simulink model "modello_adattativo"  (R2024a)
settings: Solver=VariableStepAuto  StartTime=0.0  StopTime=70  RelTol=1e-3
model workspace (MAT data in the model file):
  q0 = [0.785398163397; 0.523598775598; 0.628318530718; 0.5]
values from neighbouring files (symbols this model uses):
  Kd = diag([108 68 58 200])    [TRAIETTORIA.m]    (also in traiettoriafperfettadefinitiva1.m)
  Kp = diag([13 13 11 1000])    [TRAIETTORIA.m]    (also in traiettoriafperfettadefinitiva1.m)
  PI0 = [ml1; Il1; Im1; Fm1; ml2; Il2; Im2; Fm2; ml3; Im3; Fm3;ml4; Il4; Im4; Fm4]    [traiettoriafperfettadefinitiva1.m]
undefined symbols (not defined in the file or in its folder): DiscIntNeverNeededParam
settings Model: Creator=ThinkPad  LastModifiedBy=UTENTE
settings ModelReferenceCC: EnableRefExpFcnMdlSchedulingChecks=on
settings RTWCC: GPUComputeCapability=3.5

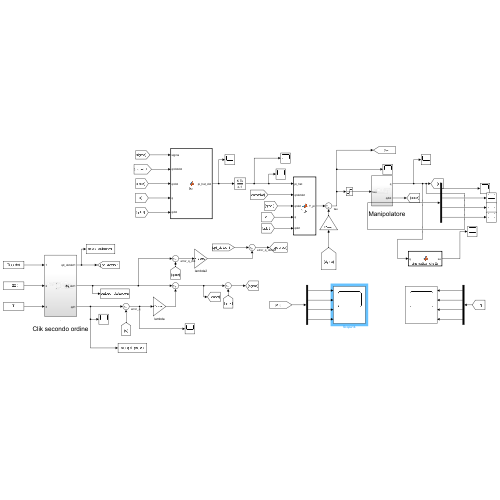
[thumbnail: Simulink's stored preview of the top-level diagram]
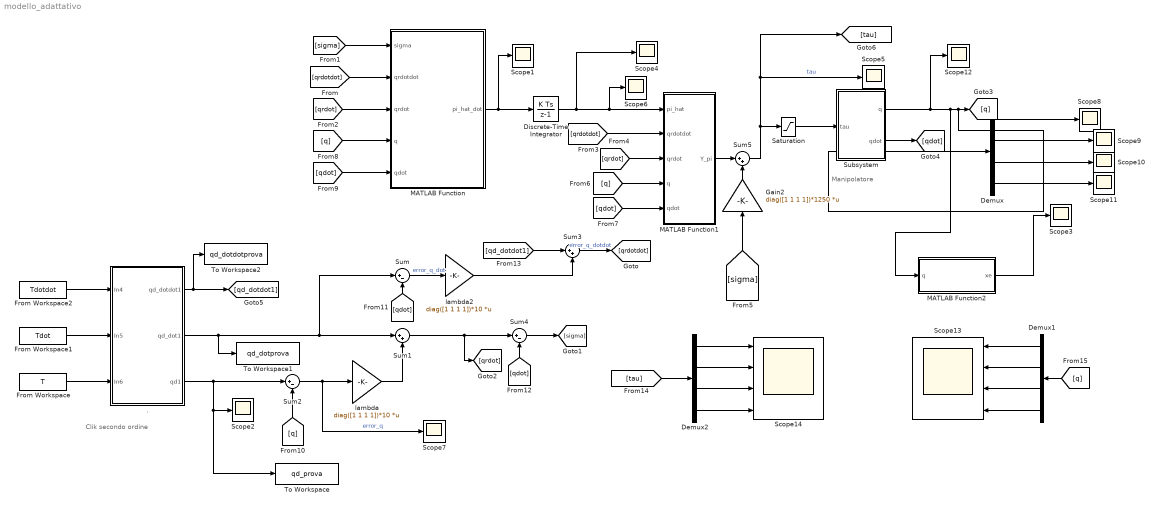
== system modello_adattativo ==
  note: Clik secondo ordine
  note: Manipolatore
  . : Subsystem
  Demux : Demux
  Demux1 : Demux
  Demux2 : Demux
  Discrete-Time Integrator : DiscreteIntegrator  InitialCondition=PI0  SampleTime=0.001  ICPrevOutput=DiscIntNeverNeededParam  ICPrevScaledInput=DiscIntNeverNeededParam
  From Workspace : FromWorkspace  VariableName=T  SampleTime=0.001
  From Workspace1 : FromWorkspace  VariableName=Tdot  SampleTime=0.001
  From Workspace2 : FromWorkspace  VariableName=Tdotdot  SampleTime=0.001
  Gain2 : Gain  Gain=diag([1 1 1 1])*1250  Multiplication=Matrix(K*u) (u vector)
  MATLAB Function : MATLAB Function  TreatAsAtomicUnit=on
  MATLAB Function1 : MATLAB Function  TreatAsAtomicUnit=on
  MATLAB Function2 : MATLAB Function  TreatAsAtomicUnit=on
  Saturation : Saturate  UpperLimit=1000  LowerLimit=-1000
  Scope{1..12} (12 alike) : Scope
  Scope13 : Scope  NumInputPorts=4
  Scope14 : Scope  NumInputPorts=4
  Subsystem : Subsystem
  Sum : Sum  Inputs=|+-
  Sum1 : Sum  Inputs=|++
  Sum2 : Sum  Inputs=|+-
  Sum3 : Sum  Inputs=|++
  Sum4 : Sum  Inputs=|+-
  Sum5 : Sum  Inputs=|++
  To Workspace : ToWorkspace  VariableName=qd_prova  SampleTime=0.001
  To Workspace1 : ToWorkspace  VariableName=qd_dotprova  SampleTime=0.001
  To Workspace2 : ToWorkspace  VariableName=qd_dotdotprova  SampleTime=0.001
  lambda : Gain  Gain=diag([1 1 1 1])*10  Multiplication=Matrix(K*u) (u vector)
  lambda2 : Gain  Gain=diag([1 1 1 1])*10  Multiplication=Matrix(K*u) (u vector)
  wires:
  From Workspace/1 -> ./3(In6)
  Subsystem/1(q) -> Scope12/1, MATLAB Function2/1(q), Demux/1, [q]
  [sigma] -> Gain2/1
  Demux2/3 -> Scope14/3
  Demux2/4 -> Scope14/4
  MATLAB Function1/1(Y_pi) -> Sum5/1
  Demux1/3 -> Scope13/3
  [q] -> MATLAB Function/4(q)
  Demux2/2 -> Scope14/2
  [qdot] -> Sum/2
  Demux1/2 -> Scope13/2
  Demux1/4 -> Scope13/4
  [qdot] -> MATLAB Function/5(qdot)
  Demux1/1 -> Scope13/1
  [sigma] -> MATLAB Function/1(sigma)
  [qdot] -> Sum4/2
  ./3(qd1) -> To Workspace/1, Scope2/1, Sum2/1
  Demux/3 -> Scope10/1
  Sum1/1 -> Sum4/1, [qrdot]
  [qrdotdot] -> MATLAB Function1/2(qrdotdot)
  [qrdotdot] -> MATLAB Function/2(qrdotdot)
  Demux2/1 -> Scope14/1
  Demux/2 -> Scope9/1
  Sum3/1 -> [qrdotdot]  "error_q_dotdot"
  Discrete-Time Integrator/1 -> Scope4/1, Scope6/1, MATLAB Function1/1(pi_hat)
  From Workspace2/1 -> ./1(In4)
  MATLAB Function2/1(xe) -> Scope3/1
  [q] -> Sum2/2
  [qdot] -> MATLAB Function1/5(qdot)
  From Workspace1/1 -> ./2(In5)
  Sum2/1 -> lambda/1, Scope7/1  "error_q"
  lambda2/1 -> Sum3/2
  Gain2/1 -> Sum5/2
  Sum5/1 -> Saturation/1, [tau], Scope5/1  "tau"
  MATLAB Function/1(pi_hat_dot) -> Discrete-Time Integrator/1, Scope1/1
  [qrdot] -> MATLAB Function/3(qrdot)
  Sum4/1 -> [sigma]
  ./1(qd_dotdot1) -> To Workspace2/1, [qd_dotdot1]
  Demux/4 -> Scope11/1
  Subsystem/2(qdot) -> [qdot]
  Sum/1 -> lambda2/1  "error_q_dot"
  [q] -> MATLAB Function1/4(q)
  lambda/1 -> Sum1/2
  ./2(qd_dot1) -> To Workspace1/1, Sum/1, Sum1/1
  Demux/1 -> Scope8/1
  [qrdot] -> MATLAB Function1/3(qrdot)
  [qd_dotdot1] -> Sum3/1
  [tau] -> Demux2/1
  [q] -> Demux1/1
  Saturation/1 -> Subsystem/1(tau)

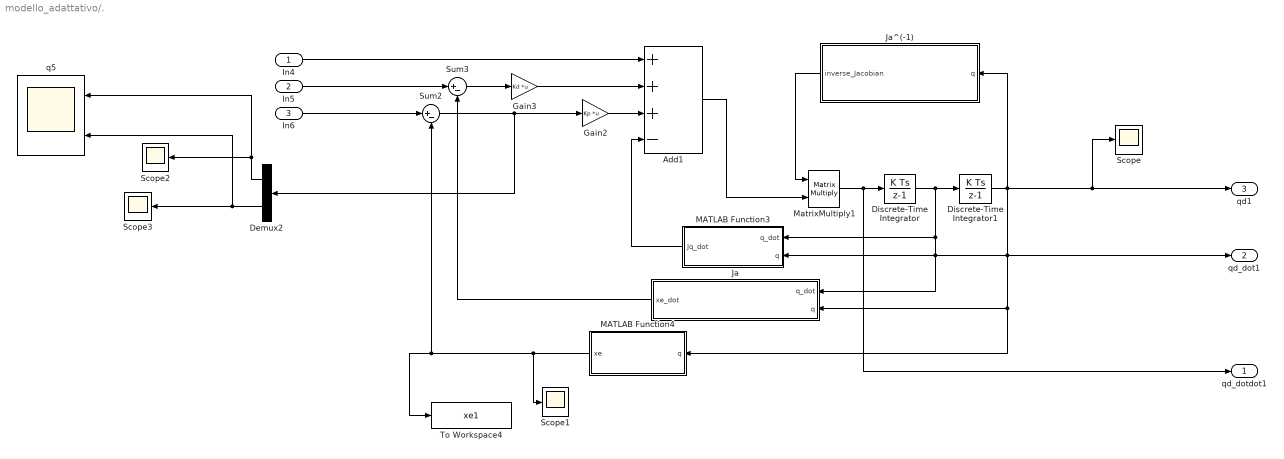
== system modello_adattativo/. ==
  In4 : Inport
  In5 : Inport  Port=2
  In6 : Inport  Port=3
  Add1 : Sum  Inputs=+++-
  Demux2 : Demux  Outputs=[3 1]
  Discrete-Time Integrator : DiscreteIntegrator  InitialCondition=[0 0 0 0]'  SampleTime=0.001  ICPrevOutput=DiscIntNeverNeededParam  ICPrevScaledInput=DiscIntNeverNeededParam
  Discrete-Time Integrator1 : DiscreteIntegrator  InitialCondition=q0  SampleTime=0.001  ICPrevOutput=DiscIntNeverNeededParam  ICPrevScaledInput=DiscIntNeverNeededParam
  Gain2 : Gain  Gain=Kp  Multiplication=Matrix(K*u)
  Gain3 : Gain  Gain=Kd  Multiplication=Matrix(K*u)
  Ja : MATLAB Function  TreatAsAtomicUnit=on
  Ja^(-1) : MATLAB Function  TreatAsAtomicUnit=on
  MATLAB Function3 : MATLAB Function  TreatAsAtomicUnit=on
  MATLAB Function4 : MATLAB Function  TreatAsAtomicUnit=on
  MatrixMultiply1 : Product  Multiplication=Matrix(*)
  Scope{,1..3} (4 alike) : Scope
  Sum2 : Sum  Inputs=|+-
  Sum3 : Sum  Inputs=|+-
  To Workspace4 : ToWorkspace  VariableName=xe1  SampleTime=0.001
  q5 : Scope  NumInputPorts=2
  qd_dotdot1 : Outport
  qd_dot1 : Outport  Port=2
  qd1 : Outport  Port=3
  wires:
  Discrete-Time Integrator1/1 -> Scope/1, qd1/1, Ja/2(q), MATLAB Function4/1(q), MATLAB Function3/2(q), Ja^(-1)/1(q)
  MatrixMultiply1/1 -> qd_dotdot1/1, Discrete-Time Integrator/1
  Sum3/1 -> Gain3/1
  MATLAB Function3/1(Jq_dot) -> Add1/4
  Ja/1(xe_dot) -> Sum3/2
  Ja^(-1)/1(inverse_Jacobian) -> MatrixMultiply1/1
  Add1/1 -> MatrixMultiply1/2
  MATLAB Function4/1(xe) -> Scope1/1, To Workspace4/1, Sum2/2
  Discrete-Time Integrator/1 -> Ja/1(q_dot), qd_dot1/1, MATLAB Function3/1(q_dot), Discrete-Time Integrator1/1
  Gain3/1 -> Add1/2
  In4/1 -> Add1/1
  In6/1 -> Sum2/1
  In5/1 -> Sum3/1
  Gain2/1 -> Add1/3
  Demux2/2 -> q5/2, Scope3/1
  Sum2/1 -> Demux2/1, Gain2/1
  Demux2/1 -> q5/1, Scope2/1

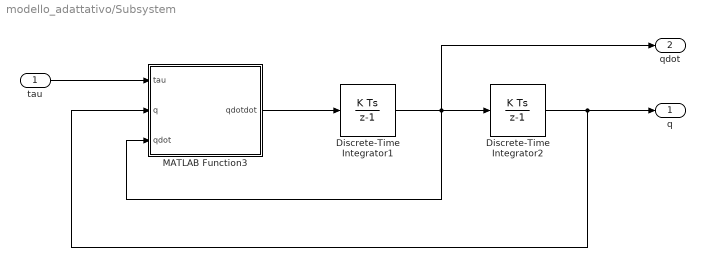
== system modello_adattativo/Subsystem ==
  tau : Inport
  Discrete-Time Integrator1 : DiscreteIntegrator  InitialCondition=[0 0 0 0]'  SampleTime=0.001  ICPrevOutput=DiscIntNeverNeededParam  ICPrevScaledInput=DiscIntNeverNeededParam
  Discrete-Time Integrator2 : DiscreteIntegrator  InitialCondition=[pi/4,pi/6,pi/5,0.5]'  SampleTime=0.001  ICPrevOutput=DiscIntNeverNeededParam  ICPrevScaledInput=DiscIntNeverNeededParam
  MATLAB Function3 : MATLAB Function  TreatAsAtomicUnit=on
  q : Outport
  qdot : Outport  Port=2
  wires:
  Discrete-Time Integrator2/1 -> q/1, MATLAB Function3/2(q)
  Discrete-Time Integrator1/1 -> qdot/1, Discrete-Time Integrator2/1, MATLAB Function3/3(qdot)
  tau/1 -> MATLAB Function3/1(tau)
  MATLAB Function3/1(qdotdot) -> Discrete-Time Integrator1/1

== matlab function modello_adattativo/Subsystem/MATLAB Function3 ==
  data: tau input; q input; qdot input; qdotdot output
function qdotdot = fcn(tau, q, qdot)
    d0=1; %m
    a1=0.5; %m
    a2=0.5; %m
    
    l1=0.25; %m
    l2=0.25; %m
    ml1=20; %kg
    ml2=20; %kg
    ml3=10; %kg
    ml4=0; %kg
    Il1=4; %kg�m2
    Il2=4; %kg�m2
    Il3=0;
    Il4=1; %kg�m2
    Kr1=1;
    Kr2=1;
    Kr3=50; %rad/m
    Kr4 =20;
    Im1=0.01; %kg�m2
    Im2=0.01; %kg�m2
    Im3=0.005; %kg�m2
    Im4=0.001;%kg
    Fm1=0.00005; %N�m�s/rad
    Fm2=0.00005; %N�m�s/rad
    Fm3=0.01; %N�m�s/rad
    Fm4 =0.005; %N�m�s/rad
    mm1=0;
    mm2=0;
    mm3=0;
    mm4=0;
    ml=3;
    
    Jp_l1=[-l1*sin(q(1)) 0 0 0; 
            l1*cos(q(1)) 0 0 0; 
            0 0 0 0];
    Jo_l1=[zeros(2,4)
           1 0 0 0];
    
    Jp_l2=[-a1*sin(q(1))-l2*sin(q(1)+q(2)) -l2*sin(q(1)+q(2)) 0 0; 
            a1*cos(q(1))+l2*cos(q(1)+q(2)) l2*cos(q(1)+q(2)) 0 0;
            0 0 0 0];
    Jo_l2=[zeros(2,4)
           1 1 0 0];
    
    Jp_l3=[-a1*sin(q(1))-a2*sin(q(1)+q(2)) -a2*sin(q(1)+q(2)) 0 0; 
            a1*cos(q(1))+a2*cos(q(1)+q(2)) a2*cos(q(1)+q(2)) 0 0;
            0 0 -1 0];
    Jo_l3 = [zeros(2,4)
             1 1 0 0];
    
    Jp_l4=Jp_l3;
    Jo_l4 = [zeros(2,4)
             1 1 0 -1];
    
    Jp_m1 = [0 0 0 0;
             0 0 0 0;
             0 0 0 0];
    Jo_m1 = [zeros(2,4)
             Kr1 0 0 0];
    
    Jp_m2 = [-a1*sin(q(1)) 0 0 0; 
            a1*cos(q(1)) 0 0 0; 
            0 0 0 0];
    Jo_m2 = [zeros(2,4)
             1 Kr2 0 0];
    
    Jp_m3 = [-a1*sin(q(1))-a2*sin(q(1)+q(2)) -a2*sin(q(1)+q(2)) 0 0; 
              a1*cos(q(1))+a2*cos(q(1)+q(2)) a2*cos(q(1)+q(2)) 0 0;
              0 0 0 0];
    Jo_m3 = [zeros(2,4)
             1 1 -Kr3 0];
    
    Jp_m4 = [-a1*sin(q(1))-a2*sin(q(1)+q(2)) -a2*sin(q(1)+q(2)) 0 0; 
              a1*cos(q(1))+a2*cos(q(1)+q(2)) a2*cos(q(1)+q(2)) 0 0;
              0 0 -1 0];
    Jo_m4 = [zeros(2,4)
             1 1 0 -Kr4];
    B1 = ml1*Jp_l1'*Jp_l1+Jo_l1'*Il1*Jo_l1+mm1*Jp_m1'*Jp_m1+Jo_m1'*Im1*Jo_m1;
    B2 = ml2*Jp_l2'*Jp_l2+Jo_l2'*Il2*Jo_l2+mm2*Jp_m2'*Jp_m2+Jo_m2'*Im2*Jo_m2;
    B3 = ml3*Jp_l3'*Jp_l3+Jo_l3'*Il3*Jo_l3+mm3*Jp_m3'*Jp_m3+Jo_m3'*Im3*Jo_m3;
    B4 = (ml4+ml)*Jp_l4'*Jp_l4+Jo_l4'*Il4*Jo_l4+mm4*Jp_m4'*Jp_m4+Jo_m4'*Im4*Jo_m4;
    B = B1+B2+B3+B4;
    
    Fv = diag([Kr1^2*Fm1 Kr2^2*Fm2 Kr3^2*Fm3 Kr4^2*Fm4]);
    g=[0 0 -9.81*(ml+ml3) 0]';
    
Jpl1_dq1=[-l1*cos(q(1)) 0 0 0;
    -l1*sin(q(1)) 0 0 0;
    0 0 0 0];

Jpl2_dq1=[-a1*cos(q(1))-l2*cos(q(1)+q(2)) -l2*cos(q(1)+q(2)) 0 0;
    -a1*sin(q(1))-l2*sin(q(1)+q(2)) -l2*sin(q(1)+q(2)) 0 0;
    0 0 0 0];

Jpl2_dq2=[-a2*cos(q(1)+q(2)) -a2*cos(q(1)+q(2)) 0 0;
    -a2*sin(q(1)+q(2)) -a2*sin(q(1)+q(2)) 0 0;
    0 0 0 0];

Jpl4_dq1=[-a1*cos(q(1))-a2*cos(q(1)+q(2)) -a2*cos(q(1)+q(2)) 0 0;
    -a1*sin(q(1))-a2*sin(q(1)+q(2)) -a2*sin(q(1)+q(2)) 0 0;
    0 0 0 0];

Jpl4_dq2=[-a2*sin(q(1)+q(2)) -a2*sin(q(1)+q(2)) 0 0;
    -a2*cos(q(1)+q(2)) -a2*cos(q(1)+q(2)) 0 0;
    0 0 0 0];

% Calcolo matrice differenziate rispetto a dq1 dq2
dBdq1=ml1*(Jpl1_dq1'*Jp_l1+Jp_l1'*Jpl1_dq1)+ml2*(Jpl2_dq1'*Jp_l2+Jp_l2'*Jpl2_dq1)...
    +ml3*(Jpl4_dq1'*Jp_l4+Jp_l4'*Jpl4_dq1);

dBdq2=ml2*(Jpl2_dq2'*Jp_l2+Jp_l2'*Jpl2_dq2)+ml3*(Jpl4_dq2'*Jp_l4+Jp_l4'*Jpl4_dq2);

H=zeros(4,4,4);

% Inizializzazione simboli cristoffel del primo tipo
for i=1:4
    for j=1:4
        for k=1:4
            H(i,j,k)=0;
        end
    end
end

H(1,1,2)=1/2*(dBdq2(1,1)+dBdq1(1,2)-dBdq1(1,2));
H(1,2,1)=H(1,1,2); 
H(1,2,2)=1/2*(dBdq2(1,2)+dBdq2(1,2)-dBdq1(2,2));
H(2,1,1)=1/2*(dBdq1(2,1)+dBdq1(2,1)-dBdq2(1,1));
H(2,1,2)=1/2*(dBdq2(2,1)+dBdq1(2,2)-dBdq2(1,2));
H(2,2,1)=H(2,1,2);
H(2,2,2)=1/2*(dBdq2(2,2)+dBdq2(2,2)-dBdq2(2,2));


% C=sym('C',[4,4]);
C=zeros(4,4);
for i=1:4
    for j=1:4
        C(i,j)=0;
    end
end

% qdot=sym('qdot',[4,1]);

for i=1:4
    for j=1:4
        for k=1:4
            r=H(i,j,k)*qdot(k);
            C(i,j)=C(i,j)+r;
        end
    end
end

    
qdotdot = inv(B)*(tau-C*qdot-Fv*qdot-g);
end

== matlab function modello_adattativo/MATLAB Function ==
  data: sigma input; qrdotdot input; qrdot input; pi_hat_dot output; q input; qdot input
function pi_hat_dot = fcn(sigma, qrdotdot,qrdot,q,qdot)

d0=1; 
a1=0.5; 
a2=0.5;    
l1=0.25;
l2=0.25;
ml1=20; 
ml2=20; 
ml3=10; 
ml4=0; 
Il1=4; 
Il2=4; 
Il3=0;
Il4=1; 
kr1=1;
kr2=1;
kr3=50;
kr4 =20;
Im1=0.01;
Im2=0.01;
Im3=0.005;
Im4=0.001;
Fm1=0.00005;
Fm2=0.00005;
Fm3=0.01;
Fm4 =0.005;
mm1=0;
mm2=0;
mm3=0;
mm4=0;
ml=3;
    
pi = [ml1; Il1; Im1; Fm1; ml2; Il2; Im2; Fm2; ml3; Im3; Fm3;ml4; Il4; Im4; Fm4];
%Kpi=diag([650 500 500 500 650 500 150 500 200 850 200 0.1 650 1500 650]);

%Kpi=diag([3000 3000 3000 3000 3000 3000 3000 300 100 100 100 0.01 300 300 300]);
%Kpi=diag([1 1 1 1 1 1 1 1 1 1 1 0.01 1 1 1]*50);
Kpi=diag([500 500 500 500 500 500 500 500 500 50 500 0.01 500 500 500]);

qr1_dd = qrdotdot(1);
qr2_dd = qrdotdot(2);
qr3_dd = qrdotdot(3);
qr4_dd = qrdotdot(4);
qr1_d = qrdot(1);
qr2_d = qrdot(2);
qr3_d = qrdot(3);
qr4_d = qrdot(4);
q1 = q(1);
q2 = q(2);
q1_d = qdot(1);
q2_d = qdot(2);

% Y =[qrdotdot(1)*((cos(conj(q(1)))*cos(q(1)))/16 + (sin(conj(q(1)))*sin(q(1)))/16), qrdotdot(1), qrdotdot(1), qrdot(1), qrdotdot(2)*(cos(q(1) + q(2) - conj(q(1)) - conj(q(2)))/16 + cos(q(1) + q(2) - conj(q(1)))/8) + qrdotdot(1)*((cos(q(1) + q(2))/4 + cos(q(1))/2)*(cos(conj(q(1)))/2 + cos(conj(q(1)) + conj(q(2)))/4) + (sin(q(1) + q(2))/4 + sin(q(1))/2)*(sin(conj(q(1)))/2 + sin(conj(q(1)) + conj(q(2)))/4)), qrdotdot(1) + qrdotdot(2), qrdotdot(1) + qrdotdot(2), 0, qrdotdot(2)*(cos(q(1) + q(2) - conj(q(1)) - conj(q(2)))/4 + cos(q(1) + q(2) - conj(q(1)))/4) + qrdotdot(1)*((cos(q(1) + q(2))/2 + cos(q(1))/2)*(cos(conj(q(1)))/2 + cos(conj(q(1)) + conj(q(2)))/2) + (sin(q(1) + q(2))/2 + sin(q(1))/2)*(sin(conj(q(1)))/2 + sin(conj(q(1)) + conj(q(2)))/2)), qrdotdot(1) + qrdotdot(2) - 50*qrdotdot(3), 0, qrdotdot(1) + qrdotdot(2) - qrdotdot(4), qrdotdot(1) + qrdotdot(2) - 20*qrdotdot(4), 0;
% 0, 0, 0, 0, qrdotdot(1)*((cos(conj(q(1)) + conj(q(2)))*(cos(q(1) + q(2))/4 + cos(q(1))/2))/4 + (sin(conj(q(1)) + conj(q(2)))*(sin(q(1) + q(2))/4 + sin(q(1))/2))/4) + (qrdotdot(2)*cos(q(1) + q(2) - conj(q(1)) - conj(q(2))))/16, qrdotdot(1) + qrdotdot(2), qrdotdot(1) + qrdotdot(2), qrdot(2), qrdotdot(1)*((cos(conj(q(1)) + conj(q(2)))*(cos(q(1) + q(2))/2 + cos(q(1))/2))/2 + (sin(conj(q(1)) + conj(q(2)))*(sin(q(1) + q(2))/2 + sin(q(1))/2))/2) + (qrdotdot(2)*cos(q(1) + q(2) - conj(q(1)) - conj(q(2))))/4, qrdotdot(1) + qrdotdot(2) - 50*qrdotdot(3), 0, qrdotdot(1) + qrdotdot(2) - qrdotdot(4), qrdotdot(1) + qrdotdot(2) - 20*qrdotdot(4), 0;
% 0, 0, 0, 0, 0, 0, 0, 0, qrdotdot(3) - 981/100, 2500*qrdotdot(3) - 50*qrdotdot(2) - 50*qrdotdot(1), 2500*qrdot(3), 0, 0, 0;
% 0, 0, 0, 0, 0, 0, 0, 0, 0, 0, 0, qrdotdot(4) - qrdotdot(2) - qrdotdot(1), 400*qrdotdot(4) - 20*qrdotdot(2) - 20*qrdotdot(1), 400*qrdot(4)];
 

% Y =[l1^2*qrdotdot(1)*cos(q(1) - conj(q(1))), qrdotdot(1), kr1^2*qrdotdot(1), kr1^2*qrdot(1), l2^2*qrdotdot(1)*cos(q(1) + q(2) - conj(q(1)) - conj(q(2))) + l2^2*qrdotdot(2)*cos(q(1) + q(2) - conj(q(1)) - conj(q(2))) + a1^2*qrdotdot(1)*cos(q(1) - conj(q(1))) + a1*l2*qrdotdot(1)*cos(q(1) + q(2) - conj(q(1))) + a1*l2*qrdotdot(2)*cos(q(1) + q(2) - conj(q(1))) - (a1*a2*qrdot(2)*sin(q(1) + q(2) - conj(q(1))))/2 + a1*l2*qrdotdot(1)*cos(conj(q(1)) - q(1) + conj(q(2))) - (a1*a2*qrdot(2)*sin(conj(q(1)) - q(1) + conj(q(2))))/2, qrdotdot(1) + qrdotdot(2),       qrdotdot(1) + kr2*qrdotdot(2),            0, a2^2*qrdotdot(1)*cos(q(1) + q(2) - conj(q(1)) - conj(q(2))) - a2^2*qrdot(2)*cos(2*real(q(1)) + 2*real(q(2))) + a2^2*qrdotdot(2)*cos(q(1) + q(2) - conj(q(1)) - conj(q(2))) + a1^2*qrdotdot(1)*cos(q(1) - conj(q(1))) - (a1*a2*qrdot(2)*cos(2*real(q(1)) + conj(q(2))))/2 + a1*a2*qrdotdot(1)*cos(q(1) + q(2) - conj(q(1))) + a1*a2*qrdotdot(2)*cos(q(1) + q(2) - conj(q(1))) + a1*a2*qrdotdot(1)*cos(conj(q(1)) - q(1) + conj(q(2))) - (a1*a2*qrdot(2)*cos(q(2) + 2*real(q(1))))/2,           qrdotdot(1) + qrdotdot(2) - kr3*qrdotdot(3),            0, qrdotdot(1) + qrdotdot(2) - qrdotdot(4),           qrdotdot(1) + qrdotdot(2) - kr4*qrdotdot(4),            0;
%                                 0,         0,               0,            0,                                                                                                                                                                                                                     l2^2*qrdotdot(1)*cos(q(1) + q(2) - conj(q(1)) - conj(q(2))) + l2^2*qrdotdot(2)*cos(q(1) + q(2) - conj(q(1)) - conj(q(2))) + a1*l2*qrdotdot(1)*cos(conj(q(1)) - q(1) + conj(q(2))), qrdotdot(1) + qrdotdot(2), qrdotdot(2)*kr2^2 + qrdotdot(1)*kr2, kr2^2*qrdot(2),                                                                                                                                                                                                                                                          a2^2*qrdotdot(1)*cos(q(1) + q(2) - conj(q(1)) - conj(q(2))) + a2^2*qrdotdot(2)*cos(q(1) + q(2) - conj(q(1)) - conj(q(2))) + a1*a2*qrdotdot(1)*cos(conj(q(1)) - q(1) + conj(q(2))),           qrdotdot(1) + qrdotdot(2) - kr3*qrdotdot(3),            0, qrdotdot(1) + qrdotdot(2) - qrdotdot(4),           qrdotdot(1) + qrdotdot(2) - kr4*qrdotdot(4),            0;
%                                 0,         0,               0,            0,                                                                                                                                                                                                                                                                                                                                                                         0,                     0,                               0,            0,                                                                                                                                                                                                                                                                                                                                                                                            qrdotdot(3) - 981/100, kr3^2*qrdotdot(3) - kr3*qrdotdot(2) - kr3*qrdotdot(1), kr3^2*qrdot(3),                                 0,                                               0,            0;
%                                0,         0,               0,            0,                                                                                                                                                                                                                                                                                                                                                                         0,                     0,                               0,            0,                                                                                                                                                                                                                                                                                                                                                                                                              0,                                               0,            0, qrdotdot(4) - qrdotdot(2) - qrdotdot(1), kr4^2*qrdotdot(4) - kr4*qrdotdot(2) - kr4*qrdotdot(1), kr4^2*qrdot(4)];
%  
Y= [qr1_dd*(cos(q1)^2/16 + sin(q1)^2/16), qr1_dd, qr1_dd, qr1_d, qr1_dd*((sin(q1 + q2)/4 + sin(q1)/2)^2 + (cos(q1 + q2)/4 + cos(q1)/2)^2) - qr2_d*(q1_d*((sin(q1 + q2)*(cos(q1 + q2)/4 + cos(q1)/2))/2 - (cos(q1 + q2)*(sin(q1 + q2)/4 + sin(q1)/2))/2) + q2_d*((sin(q1 + q2)*(cos(q1 + q2)/4 + cos(q1)/2))/2 - (cos(q1 + q2)*(sin(q1 + q2)/4 + sin(q1)/2))/2)) + qr2_dd*((cos(q1 + q2)*(cos(q1 + q2)/4 + cos(q1)/2))/4 + (sin(q1 + q2)*(sin(q1 + q2)/4 + sin(q1)/2))/4) - q1_d*qr1_d*((sin(q1 + q2)*(cos(q1 + q2)/4 + cos(q1)/2))/2 - (cos(q1 + q2)*(sin(q1 + q2)/4 + sin(q1)/2))/2), qr1_dd + qr2_dd, qr1_dd + qr2_dd,     0, qr1_dd*((sin(q1 + q2)/2 + sin(q1)/2)^2 + (cos(q1 + q2)/2 + cos(q1)/2)^2) - qr2_d*(q2_d*(cos(q1 + q2)^2/4 - sin(q1 + q2)^2/4 + (cos(q1 + q2)*(cos(q1 + q2)/2 + cos(q1)/2))/2 - (sin(q1 + q2)*(sin(q1 + q2)/2 + sin(q1)/2))/2) + q1_d*((cos(q1 + q2)*(cos(q1 + q2)/2 + cos(q1)/2))/2 - (sin(q1 + q2)*(sin(q1 + q2)/2 + sin(q1)/2))/2)) + qr2_dd*((cos(q1 + q2)*(cos(q1 + q2)/2 + cos(q1)/2))/2 + (sin(q1 + q2)*(sin(q1 + q2)/2 + sin(q1)/2))/2) - q1_d*qr1_d*((cos(q1 + q2)*(cos(q1 + q2)/2 + cos(q1)/2))/2 - (sin(q1 + q2)*(sin(q1 + q2)/2 + sin(q1)/2))/2),         qr1_dd + qr2_dd - 50*qr3_dd,          0, qr1_dd*((sin(q1 + q2)/2 + sin(q1)/2)^2 + (cos(q1 + q2)/2 + cos(q1)/2)^2) + qr2_dd*((cos(q1 + q2)*(cos(q1 + q2)/2 + cos(q1)/2))/2 + (sin(q1 + q2)*(sin(q1 + q2)/2 + sin(q1)/2))/2), qr1_dd + qr2_dd - qr4_dd,        qr1_dd + qr2_dd - 20*qr4_dd,         0
                                   0,      0,      0,     0,                                                                                                                                                                                                                                                 qr2_dd*(cos(q1 + q2)^2/16 + sin(q1 + q2)^2/16) + qr1_dd*((cos(q1 + q2)*(cos(q1 + q2)/4 + cos(q1)/2))/4 + (sin(q1 + q2)*(sin(q1 + q2)/4 + sin(q1)/2))/4) + q1_d*qr1_d*((sin(q1 + q2)*(cos(q1 + q2)/4 + cos(q1)/2))/2 - (cos(q1 + q2)*(sin(q1 + q2)/4 + sin(q1)/2))/2), qr1_dd + qr2_dd, qr1_dd + qr2_dd, qr2_d,                                                                                                                                                                                                                                  qr2_dd*(cos(q1 + q2)^2/4 + sin(q1 + q2)^2/4) + qr1_dd*((cos(q1 + q2)*(cos(q1 + q2)/2 + cos(q1)/2))/2 + (sin(q1 + q2)*(sin(q1 + q2)/2 + sin(q1)/2))/2) + q1_d*qr1_d*((cos(q1 + q2)*(cos(q1 + q2)/2 + cos(q1)/2))/2 - (sin(q1 + q2)*(sin(q1 + q2)/2 + sin(q1)/2))/2) - (q2_d*qr2_d*(cos(q1 + q2)^2/2 - sin(q1 + q2)^2/2))/2,         qr1_dd + qr2_dd - 50*qr3_dd,          0,                             qr2_dd*(cos(q1 + q2)^2/4 + sin(q1 + q2)^2/4) + qr1_dd*((cos(q1 + q2)*(cos(q1 + q2)/2 + cos(q1)/2))/2 + (sin(q1 + q2)*(sin(q1 + q2)/2 + sin(q1)/2))/2), qr1_dd + qr2_dd - qr4_dd,        qr1_dd + qr2_dd - 20*qr4_dd,         0
                                  0,      0,      0,     0,                                                                                                                                                                                                                                                                                                                                                                                                                                                                                                                    0,               0,               0,     0,                                                                                                                                                                                                                                                                                                                                                                                                                                                                                                                                           qr3_dd - 981/100, 2500*qr3_dd - 50*qr2_dd - 50*qr1_dd, 2500*qr3_d,                                                                                                                                                                            qr3_dd,                        0,                                  0,         0
                                   0,      0,      0,     0,                                                                                                                                                                                                                                                                                                                                                                                                                                                                                                                    0,               0,               0,     0,                                                                                                                                                                                                                                                                                                                                                                                                                                                                                                                                                          0,                                   0,          0,                                                                                                                                                                                 0, qr4_dd - qr2_dd - qr1_dd, 400*qr4_dd - 20*qr2_dd - 20*qr1_dd, 400*qr4_d];

% Y = ones(4,15);

% Y = [qr1_dd*(cos(q1)^2/16 + sin(q1)^2/16), qr1_dd, qr1_dd, qr1_d, qr1_dd*((sin(q1 + q2)/4 + sin(q1)/2)^2 + (cos(q1 + q2)/4 + cos(q1)/2)^2) + qr2_dd*((cos(q1 + q2)*(cos(q1 + q2)/4 + cos(q1)/2))/4 + (sin(q1 + q2)*(sin(q1 + q2)/4 + sin(q1)/2))/4), qr1_dd + qr2_dd, qr1_dd + qr2_dd,     0, qr1_dd*((sin(q1 + q2)/2 + sin(q1)/2)^2 + (cos(q1 + q2)/2 + cos(q1)/2)^2) + qr2_dd*((cos(q1 + q2)*(cos(q1 + q2)/2 + cos(q1)/2))/2 + (sin(q1 + q2)*(sin(q1 + q2)/2 + sin(q1)/2))/2),         qr1_dd + qr2_dd - 50*qr3_dd,          0, qr1_dd*((sin(q1 + q2)/2 + sin(q1)/2)^2 + (cos(q1 + q2)/2 + cos(q1)/2)^2) + qr2_dd*((cos(q1 + q2)*(cos(q1 + q2)/2 + cos(q1)/2))/2 + (sin(q1 + q2)*(sin(q1 + q2)/2 + sin(q1)/2))/2), qr1_dd + qr2_dd - qr4_dd,        qr1_dd + qr2_dd - 20*qr4_dd,         0
%                                    0,      0,      0,     0,                           qr2_dd*(cos(q1 + q2)^2/16 + sin(q1 + q2)^2/16) + qr1_dd*((cos(q1 + q2)*(cos(q1 + q2)/4 + cos(q1)/2))/4 + (sin(q1 + q2)*(sin(q1 + q2)/4 + sin(q1)/2))/4), qr1_dd + qr2_dd, qr1_dd + qr2_dd, qr2_d,                             qr2_dd*(cos(q1 + q2)^2/4 + sin(q1 + q2)^2/4) + qr1_dd*((cos(q1 + q2)*(cos(q1 + q2)/2 + cos(q1)/2))/2 + (sin(q1 + q2)*(sin(q1 + q2)/2 + sin(q1)/2))/2),         qr1_dd + qr2_dd - 50*qr3_dd,          0,                             qr2_dd*(cos(q1 + q2)^2/4 + sin(q1 + q2)^2/4) + qr1_dd*((cos(q1 + q2)*(cos(q1 + q2)/2 + cos(q1)/2))/2 + (sin(q1 + q2)*(sin(q1 + q2)/2 + sin(q1)/2))/2), qr1_dd + qr2_dd - qr4_dd,        qr1_dd + qr2_dd - 20*qr4_dd,         0
%                                    0,      0,      0,     0,                                                                                                                                                                                 0,               0,               0,     0,                                                                                                                                                                  qr3_dd - 981/100, 2500*qr3_dd - 50*qr2_dd - 50*qr1_dd, 2500*qr3_d,                                                                                                                                                                            qr3_dd,                        0,                                  0,         0
%                                    0,      0,      0,     0,                                                                                                                                                                                 0,               0,               0,     0,                                                                                                                                                                                 0,                                   0,          0,                                                                                                                                                                                 0, qr4_dd - qr2_dd - qr1_dd, 400*qr4_dd - 20*qr2_dd - 20*qr1_dd, 400*qr4_d];
%  

pi_hat_dot=inv(Kpi)*Y'*sigma;








end

== matlab function modello_adattativo/MATLAB Function1 ==
  data: pi_hat input; Y_pi output; qrdotdot input; qrdot input; q input; qdot input
function Y_pi = Y_pi(pi_hat, qrdotdot,qrdot,q,qdot)
d0=1; 
a1=0.5; 
a2=0.5;    
l1=0.25;
l2=0.25;
ml1=20; 
ml2=20; 
ml3=10; 
ml4=0; 
Il1=4; 
Il2=4; 
Il3=0;
Il4=1; 
kr1=1;
kr2=1;
kr3=50;
kr4 =20;
Im1=0.01;
Im2=0.01;
Im3=0.005;
Im4=0.001;
Fm1=0.00005;
Fm2=0.00005;
Fm3=0.01;
Fm4 =0.005;
mm1=0;
mm2=0;
mm3=0;
mm4=0;
ml=3;


qr1_dd = qrdotdot(1);
qr2_dd = qrdotdot(2);
qr3_dd = qrdotdot(3);
qr4_dd = qrdotdot(4);
qr1_d = qrdot(1);
qr2_d = qrdot(2);
qr3_d = qrdot(3);
qr4_d = qrdot(4);
q1 = q(1);
q2 = q(2);
% q3 = q(3);
% q4 = q(4);
q1_d = qdot(1);
q2_d = qdot(2);
% 
% Y =[qrdotdot(1)*((cos(conj(q(1)))*cos(q(1)))/16 + (sin(conj(q(1)))*sin(q(1)))/16), qrdotdot(1), qrdotdot(1), qrdot(1), qrdotdot(2)*(cos(q(1) + q(2) - conj(q(1)) - conj(q(2)))/16 + cos(q(1) + q(2) - conj(q(1)))/8) + qrdotdot(1)*((cos(q(1) + q(2))/4 + cos(q(1))/2)*(cos(conj(q(1)))/2 + cos(conj(q(1)) + conj(q(2)))/4) + (sin(q(1) + q(2))/4 + sin(q(1))/2)*(sin(conj(q(1)))/2 + sin(conj(q(1)) + conj(q(2)))/4)), qrdotdot(1) + qrdotdot(2), qrdotdot(1) + qrdotdot(2), 0, qrdotdot(2)*(cos(q(1) + q(2) - conj(q(1)) - conj(q(2)))/4 + cos(q(1) + q(2) - conj(q(1)))/4) + qrdotdot(1)*((cos(q(1) + q(2))/2 + cos(q(1))/2)*(cos(conj(q(1)))/2 + cos(conj(q(1)) + conj(q(2)))/2) + (sin(q(1) + q(2))/2 + sin(q(1))/2)*(sin(conj(q(1)))/2 + sin(conj(q(1)) + conj(q(2)))/2)), qrdotdot(1) + qrdotdot(2) - 50*qrdotdot(3), 0, qrdotdot(1) + qrdotdot(2) - qrdotdot(4), qrdotdot(1) + qrdotdot(2) - 20*qrdotdot(4), 0;
% 0, 0, 0, 0, qrdotdot(1)*((cos(conj(q(1)) + conj(q(2)))*(cos(q(1) + q(2))/4 + cos(q(1))/2))/4 + (sin(conj(q(1)) + conj(q(2)))*(sin(q(1) + q(2))/4 + sin(q(1))/2))/4) + (qrdotdot(2)*cos(q(1) + q(2) - conj(q(1)) - conj(q(2))))/16, qrdotdot(1) + qrdotdot(2), qrdotdot(1) + qrdotdot(2), qrdot(2), qrdotdot(1)*((cos(conj(q(1)) + conj(q(2)))*(cos(q(1) + q(2))/2 + cos(q(1))/2))/2 + (sin(conj(q(1)) + conj(q(2)))*(sin(q(1) + q(2))/2 + sin(q(1))/2))/2) + (qrdotdot(2)*cos(q(1) + q(2) - conj(q(1)) - conj(q(2))))/4, qrdotdot(1) + qrdotdot(2) - 50*qrdotdot(3), 0, qrdotdot(1) + qrdotdot(2) - qrdotdot(4), qrdotdot(1) + qrdotdot(2) - 20*qrdotdot(4), 0;
% 0, 0, 0, 0, 0, 0, 0, 0, qrdotdot(3) - 981/100, 2500*qrdotdot(3) - 50*qrdotdot(2) - 50*qrdotdot(1), 2500*qrdot(3), 0, 0, 0;
% 0, 0, 0, 0, 0, 0, 0, 0, 0, 0, 0, qrdotdot(4) - qrdotdot(2) - qrdotdot(1), 400*qrdotdot(4) - 20*qrdotdot(2) - 20*qrdotdot(1), 400*qrdot(4)];

% Y =[l1^2*qrdotdot(1)*cos(q(1) - conj(q(1))), qrdotdot(1), kr1^2*qrdotdot(1), kr1^2*qrdot(1), l2^2*qrdotdot(1)*cos(q(1) + q(2) - conj(q(1)) - conj(q(2))) + l2^2*qrdotdot(2)*cos(q(1) + q(2) - conj(q(1)) - conj(q(2))) + a1^2*qrdotdot(1)*cos(q(1) - conj(q(1))) + a1*l2*qrdotdot(1)*cos(q(1) + q(2) - conj(q(1))) + a1*l2*qrdotdot(2)*cos(q(1) + q(2) - conj(q(1))) - (a1*a2*qrdot(2)*sin(q(1) + q(2) - conj(q(1))))/2 + a1*l2*qrdotdot(1)*cos(conj(q(1)) - q(1) + conj(q(2))) - (a1*a2*qrdot(2)*sin(conj(q(1)) - q(1) + conj(q(2))))/2, qrdotdot(1) + qrdotdot(2),       qrdotdot(1) + kr2*qrdotdot(2),            0, a2^2*qrdotdot(1)*cos(q(1) + q(2) - conj(q(1)) - conj(q(2))) - a2^2*qrdot(2)*cos(2*real(q(1)) + 2*real(q(2))) + a2^2*qrdotdot(2)*cos(q(1) + q(2) - conj(q(1)) - conj(q(2))) + a1^2*qrdotdot(1)*cos(q(1) - conj(q(1))) - (a1*a2*qrdot(2)*cos(2*real(q(1)) + conj(q(2))))/2 + a1*a2*qrdotdot(1)*cos(q(1) + q(2) - conj(q(1))) + a1*a2*qrdotdot(2)*cos(q(1) + q(2) - conj(q(1))) + a1*a2*qrdotdot(1)*cos(conj(q(1)) - q(1) + conj(q(2))) - (a1*a2*qrdot(2)*cos(q(2) + 2*real(q(1))))/2,           qrdotdot(1) + qrdotdot(2) - kr3*qrdotdot(3),            0, qrdotdot(1) + qrdotdot(2) - qrdotdot(4),           qrdotdot(1) + qrdotdot(2) - kr4*qrdotdot(4),            0;
%                                 0,         0,               0,            0,                                                                                                                                                                                                                     l2^2*qrdotdot(1)*cos(q(1) + q(2) - conj(q(1)) - conj(q(2))) + l2^2*qrdotdot(2)*cos(q(1) + q(2) - conj(q(1)) - conj(q(2))) + a1*l2*qrdotdot(1)*cos(conj(q(1)) - q(1) + conj(q(2))), qrdotdot(1) + qrdotdot(2), qrdotdot(2)*kr2^2 + qrdotdot(1)*kr2, kr2^2*qrdot(2),                                                                                                                                                                                                                                                          a2^2*qrdotdot(1)*cos(q(1) + q(2) - conj(q(1)) - conj(q(2))) + a2^2*qrdotdot(2)*cos(q(1) + q(2) - conj(q(1)) - conj(q(2))) + a1*a2*qrdotdot(1)*cos(conj(q(1)) - q(1) + conj(q(2))),           qrdotdot(1) + qrdotdot(2) - kr3*qrdotdot(3),            0, qrdotdot(1) + qrdotdot(2) - qrdotdot(4),           qrdotdot(1) + qrdotdot(2) - kr4*qrdotdot(4),            0;
%                                 0,         0,               0,            0,                                                                                                                                                                                                                                                                                                                                                                         0,                     0,                               0,            0,                                                                                                                                                                                                                                                                                                                                                                                            qrdotdot(3) - 981/100, kr3^2*qrdotdot(3) - kr3*qrdotdot(2) - kr3*qrdotdot(1), kr3^2*qrdot(3),                                 0,                                               0,            0;
%                                0,         0,               0,            0,                                                                                                                                                                                                                                                                                                                                                                         0,                     0,                               0,            0,                                                                                                                                                                                                                                                                                                                                                                                                              0,                                               0,            0, qrdotdot(4) - qrdotdot(2) - qrdotdot(1), kr4^2*qrdotdot(4) - kr4*qrdotdot(2) - kr4*qrdotdot(1), kr4^2*qrdot(4)];
%  



Y= [qr1_dd*(cos(q1)^2/16 + sin(q1)^2/16), qr1_dd, qr1_dd, qr1_d, qr1_dd*((sin(q1 + q2)/4 + sin(q1)/2)^2 + (cos(q1 + q2)/4 + cos(q1)/2)^2) - qr2_d*(q1_d*((sin(q1 + q2)*(cos(q1 + q2)/4 + cos(q1)/2))/2 - (cos(q1 + q2)*(sin(q1 + q2)/4 + sin(q1)/2))/2) + q2_d*((sin(q1 + q2)*(cos(q1 + q2)/4 + cos(q1)/2))/2 - (cos(q1 + q2)*(sin(q1 + q2)/4 + sin(q1)/2))/2)) + qr2_dd*((cos(q1 + q2)*(cos(q1 + q2)/4 + cos(q1)/2))/4 + (sin(q1 + q2)*(sin(q1 + q2)/4 + sin(q1)/2))/4) - q1_d*qr1_d*((sin(q1 + q2)*(cos(q1 + q2)/4 + cos(q1)/2))/2 - (cos(q1 + q2)*(sin(q1 + q2)/4 + sin(q1)/2))/2), qr1_dd + qr2_dd, qr1_dd + qr2_dd,     0, qr1_dd*((sin(q1 + q2)/2 + sin(q1)/2)^2 + (cos(q1 + q2)/2 + cos(q1)/2)^2) - qr2_d*(q2_d*(cos(q1 + q2)^2/4 - sin(q1 + q2)^2/4 + (cos(q1 + q2)*(cos(q1 + q2)/2 + cos(q1)/2))/2 - (sin(q1 + q2)*(sin(q1 + q2)/2 + sin(q1)/2))/2) + q1_d*((cos(q1 + q2)*(cos(q1 + q2)/2 + cos(q1)/2))/2 - (sin(q1 + q2)*(sin(q1 + q2)/2 + sin(q1)/2))/2)) + qr2_dd*((cos(q1 + q2)*(cos(q1 + q2)/2 + cos(q1)/2))/2 + (sin(q1 + q2)*(sin(q1 + q2)/2 + sin(q1)/2))/2) - q1_d*qr1_d*((cos(q1 + q2)*(cos(q1 + q2)/2 + cos(q1)/2))/2 - (sin(q1 + q2)*(sin(q1 + q2)/2 + sin(q1)/2))/2),         qr1_dd + qr2_dd - 50*qr3_dd,          0, qr1_dd*((sin(q1 + q2)/2 + sin(q1)/2)^2 + (cos(q1 + q2)/2 + cos(q1)/2)^2) + qr2_dd*((cos(q1 + q2)*(cos(q1 + q2)/2 + cos(q1)/2))/2 + (sin(q1 + q2)*(sin(q1 + q2)/2 + sin(q1)/2))/2), qr1_dd + qr2_dd - qr4_dd,        qr1_dd + qr2_dd - 20*qr4_dd,         0
                                   0,      0,      0,     0,                                                                                                                                                                                                                                                 qr2_dd*(cos(q1 + q2)^2/16 + sin(q1 + q2)^2/16) + qr1_dd*((cos(q1 + q2)*(cos(q1 + q2)/4 + cos(q1)/2))/4 + (sin(q1 + q2)*(sin(q1 + q2)/4 + sin(q1)/2))/4) + q1_d*qr1_d*((sin(q1 + q2)*(cos(q1 + q2)/4 + cos(q1)/2))/2 - (cos(q1 + q2)*(sin(q1 + q2)/4 + sin(q1)/2))/2), qr1_dd + qr2_dd, qr1_dd + qr2_dd, qr2_d,                                                                                                                                                                                                                                  qr2_dd*(cos(q1 + q2)^2/4 + sin(q1 + q2)^2/4) + qr1_dd*((cos(q1 + q2)*(cos(q1 + q2)/2 + cos(q1)/2))/2 + (sin(q1 + q2)*(sin(q1 + q2)/2 + sin(q1)/2))/2) + q1_d*qr1_d*((cos(q1 + q2)*(cos(q1 + q2)/2 + cos(q1)/2))/2 - (sin(q1 + q2)*(sin(q1 + q2)/2 + sin(q1)/2))/2) - (q2_d*qr2_d*(cos(q1 + q2)^2/2 - sin(q1 + q2)^2/2))/2,         qr1_dd + qr2_dd - 50*qr3_dd,          0,                             qr2_dd*(cos(q1 + q2)^2/4 + sin(q1 + q2)^2/4) + qr1_dd*((cos(q1 + q2)*(cos(q1 + q2)/2 + cos(q1)/2))/2 + (sin(q1 + q2)*(sin(q1 + q2)/2 + sin(q1)/2))/2), qr1_dd + qr2_dd - qr4_dd,        qr1_dd + qr2_dd - 20*qr4_dd,         0
                                  0,      0,      0,     0,                                                                                                                                                                                                                                                                                                                                                                                                                                                                                                                    0,               0,               0,     0,                                                                                                                                                                                                                                                                                                                                                                                                                                                                                                                                           qr3_dd - 981/100, 2500*qr3_dd - 50*qr2_dd - 50*qr1_dd, 2500*qr3_d,                                                                                                                                                                            qr3_dd,                        0,                                  0,         0
                                   0,      0,      0,     0,                                                                                                                                                                                                                                                                                                                                                                                                                                                                                                                    0,               0,               0,     0,                                                                                                                                                                                                                                                                                                                                                                                                                                                                                                                                                          0,                                   0,          0,                                                                                                                                                                                 0, qr4_dd - qr2_dd - qr1_dd, 400*qr4_dd - 20*qr2_dd - 20*qr1_dd, 400*qr4_d];

% Y = [qr1_dd*(cos(q1)^2/16 + sin(q1)^2/16), qr1_dd, qr1_dd, qr1_d, qr1_dd*((sin(q1 + q2)/4 + sin(q1)/2)^2 + (cos(q1 + q2)/4 + cos(q1)/2)^2) + qr2_dd*((cos(q1 + q2)*(cos(q1 + q2)/4 + cos(q1)/2))/4 + (sin(q1 + q2)*(sin(q1 + q2)/4 + sin(q1)/2))/4), qr1_dd + qr2_dd, qr1_dd + qr2_dd,     0, qr1_dd*((sin(q1 + q2)/2 + sin(q1)/2)^2 + (cos(q1 + q2)/2 + cos(q1)/2)^2) + qr2_dd*((cos(q1 + q2)*(cos(q1 + q2)/2 + cos(q1)/2))/2 + (sin(q1 + q2)*(sin(q1 + q2)/2 + sin(q1)/2))/2),         qr1_dd + qr2_dd - 50*qr3_dd,          0, qr1_dd*((sin(q1 + q2)/2 + sin(q1)/2)^2 + (cos(q1 + q2)/2 + cos(q1)/2)^2) + qr2_dd*((cos(q1 + q2)*(cos(q1 + q2)/2 + cos(q1)/2))/2 + (sin(q1 + q2)*(sin(q1 + q2)/2 + sin(q1)/2))/2), qr1_dd + qr2_dd - qr4_dd,        qr1_dd + qr2_dd - 20*qr4_dd,         0
%                                    0,      0,      0,     0,                           qr2_dd*(cos(q1 + q2)^2/16 + sin(q1 + q2)^2/16) + qr1_dd*((cos(q1 + q2)*(cos(q1 + q2)/4 + cos(q1)/2))/4 + (sin(q1 + q2)*(sin(q1 + q2)/4 + sin(q1)/2))/4), qr1_dd + qr2_dd, qr1_dd + qr2_dd, qr2_d,                             qr2_dd*(cos(q1 + q2)^2/4 + sin(q1 + q2)^2/4) + qr1_dd*((cos(q1 + q2)*(cos(q1 + q2)/2 + cos(q1)/2))/2 + (sin(q1 + q2)*(sin(q1 + q2)/2 + sin(q1)/2))/2),         qr1_dd + qr2_dd - 50*qr3_dd,          0,                             qr2_dd*(cos(q1 + q2)^2/4 + sin(q1 + q2)^2/4) + qr1_dd*((cos(q1 + q2)*(cos(q1 + q2)/2 + cos(q1)/2))/2 + (sin(q1 + q2)*(sin(q1 + q2)/2 + sin(q1)/2))/2), qr1_dd + qr2_dd - qr4_dd,        qr1_dd + qr2_dd - 20*qr4_dd,         0
%                                    0,      0,      0,     0,                                                                                                                                                                                 0,               0,               0,     0,                                                                                                                                                                  qr3_dd - 981/100, 2500*qr3_dd - 50*qr2_dd - 50*qr1_dd, 2500*qr3_d,                                                                                                                                                                            qr3_dd,                        0,                                  0,         0
%                                    0,      0,      0,     0,                                                                                                                                                                                 0,               0,               0,     0,                                                                                                                                                                                 0,                                   0,          0,                                                                                                                                                                                 0, qr4_dd - qr2_dd - qr1_dd, 400*qr4_dd - 20*qr2_dd - 20*qr1_dd, 400*qr4_d];
%  




% Y = ones(4,15);

Y_pi = Y*pi_hat;
end

== matlab function modello_adattativo/MATLAB Function2 ==
  data: q input; xe output
function xe = cinematica_diretta(q)
% T_4_0=[cos(q(4))*(cos(q(1))*cos(q(2))-sin(q1)*sin(q2))+sin(q(4))*(cos(q1)*sin(q(2))+cos(q(2))*sin(q(1)))   cos(q(4))*(cos(q(1))*sin(q(2))+cos(q(2))*sin(q(1)))-sin(q(4))*(cos(q(1))*cos(q(2))-sin(q(1))*sin(q(2)))  0 cos(q(1))/2+(cos(q(1))*cos(q(2)))/2-(sin(q(1))*sin(q(2)))/2;
%         cos(q(4))*(cos(q(1))*sin(q(2))+cos(q(2))*sin(q(1)))-sin(q(4))*(cos(q(1))*cos(q(2))-sin(q(1))*sin(q(2))) -cos(q(4))*(cos(q(1))*cos(q(2))-sin(q(1))*sin(q(2)))-sin(q(4))*(cos(q(1))*sin(q(2))+cos(q(2))*sin(q(1)))  0 sin(q(1))/2+(cos(q(1))*sin(q(2)))/2+(cos(q(2))*sin(q(2)))/2;
%                       0                                                      0                    -1                                                1-q(3);
%         0                                       0                                         0                                                                                                                                      1];

x_e=[0.5*cos(q(1))+0.5*cos(q(1)+q(2));
    0.5*sin(q(1))+0.5*sin(q(1)+q(2));
        1-q(3);
        q(1)+q(2)-q(4)];
xe=x_e;
end

== matlab function modello_adattativo/./Ja ==
  data: q_dot input; q input; xe_dot output
function xe_dot = xe_dot(q_dot, q)

J=[-0.5*sin(q(1))-0.5*sin(q(1)+q(2)) -0.5*sin(q(1)+q(2)) 0 0;
    0.5*cos(q(1))+0.5*cos(q(1)+q(2)) 0.5*cos(q(1)+q(2)) 0 0;
    0 0 -1 0;
    1 1 0 -1];
xe_dot=J*q_dot;
end

== matlab function modello_adattativo/./Ja^(-1) ==
  data: q input; inverse_Jacobian output
function inverse_Jacobian= i_j(q)

J=[-0.5*sin(q(1))-0.5*sin(q(1)+q(2)) -0.5*sin(q(1)+q(2)) 0 0;
    0.5*cos(q(1))+0.5*cos(q(1)+q(2)) 0.5*cos(q(1)+q(2)) 0 0;
    0 0 -1 0;
    1 1 0 -1];

J_inv=inv(J);

 inverse_Jacobian=J_inv;
end

== matlab function modello_adattativo/./MATLAB Function3 ==
  data: q_dot input; q input; Jq_dot output
function Jq_dot = Jq_dot(q_dot, q)
J_dot=[-0.5*cos(q(1))*q_dot(1)-0.5*cos(q(1)+q(2))*(q_dot(1)+q_dot(2)) -0.5*cos(q(1)+q(2))*(q_dot(1)+q_dot(2)) 0 0;
    -0.5*sin(q(1))*q_dot(1)-0.5*sin(q(1)+q(2))*(q_dot(1)+q_dot(2)) -0.5*sin(q(1)+q(2))*(q_dot(1)+q_dot(2)) 0 0;
    0 0 0 0;
    0 0 0 0];
Jq_dot=J_dot*q_dot;
end

== matlab function modello_adattativo/./MATLAB Function4 ==
  data: q input; xe output
function xe = cinematica_diretta(q)
% T_4_0=[cos(q(4))*(cos(q(1))*cos(q(2))-sin(q1)*sin(q2))+sin(q(4))*(cos(q1)*sin(q(2))+cos(q(2))*sin(q(1)))   cos(q(4))*(cos(q(1))*sin(q(2))+cos(q(2))*sin(q(1)))-sin(q(4))*(cos(q(1))*cos(q(2))-sin(q(1))*sin(q(2)))  0 cos(q(1))/2+(cos(q(1))*cos(q(2)))/2-(sin(q(1))*sin(q(2)))/2;
%         cos(q(4))*(cos(q(1))*sin(q(2))+cos(q(2))*sin(q(1)))-sin(q(4))*(cos(q(1))*cos(q(2))-sin(q(1))*sin(q(2))) -cos(q(4))*(cos(q(1))*cos(q(2))-sin(q(1))*sin(q(2)))-sin(q(4))*(cos(q(1))*sin(q(2))+cos(q(2))*sin(q(1)))  0 sin(q(1))/2+(cos(q(1))*sin(q(2)))/2+(cos(q(2))*sin(q(2)))/2;
%                       0                                                      0                    -1                                                1-q(3);
%         0                                       0                                         0                                                                                                                                      1];

x_e=[0.5*cos(q(1))+0.5*cos(q(1)+q(2));
    0.5*sin(q(1))+0.5*sin(q(1)+q(2));
        1-q(3);
        q(1)+q(2)-q(4)];
xe=x_e;
end
